simulink library "passive_balancing_plant_lib"  (R2022b)
settings: Solver=VariableStepAuto  StartTime=0.0  StopTime=10.0  RelTol=1e-3
values from neighbouring files (symbols this model uses):
  C1_LUT = 2887.70299486401 4322.85637783158 4303.63777361549 5660.4257619161 10025.6228486411 10795.3803188661 8403.2926645088 10303.8261927401 8639.27645423926 9127.81465902188 33086.4103910671 13371.3754375743 9514.85903729136 34662.1679971819 8026.84086107818 27790.9287411121 14186.8877450726 12734.2960214805 11929.7824894044 12691.2600304428 4549.5148639253 79281.9214895882 7004.71125363224 35331.898561    [passive_balancing_data.sldd]
  Capacity_LUT : value not decoded    [passive_balancing_data.sldd]
  cell_area = 0.1019    [passive_balancing_data.sldd]
  cell_Cp_heat = 964.92    [passive_balancing_data.sldd]
  cell_mass = 0.84    [passive_balancing_data.sldd]
  Em_LUT = 3.48407194875853 3.55418080716149 3.6044040443123 3.64321489304947 3.68502177847119 3.74422605890089 3.82967867350671 3.94315917033962 4.05943812577673 4.19049029477082 3.49373906253632 3.5525957055852 3.61410230902054 3.64896659680084 3.68864192779988 3.74398921633946 3.83940080415011 3.94854312702762 4.06094828281537 4.19030181290971 3.50592874552606 3.55508312112845 3.61515360383738 3.656857038    [passive_balancing_data.sldd]
  h_conv = 5.0    [passive_balancing_data.sldd]
  initial_SOC : value not decoded    [passive_balancing_data.sldd]
  initial_temperature = 293.15    [passive_balancing_data.sldd]
  R0_LUT = 0.0164025520353838 0.0119600956597842 0.0119853068610826 0.0111330643324705 0.011822289585725 0.0116748342939053 0.0112768580015193 0.0118933795996695 0.0120321348242062 0.0124098156482057 0.00991391593917779 0.00875043635238341 0.00832297953681552 0.00872061850253288 0.00795909444960185 0.00856548056926203 0.00843330788647423 0.00850334186162495 0.00846602435735512 0.00846539753229566 0.009331684    [passive_balancing_data.sldd]
  R1_LUT = 0.00470517937000299 0.00290275050725254 0.00173884757466172 0.00166867739185738 0.000922417169458259 0.00120601315196432 0.00134107014418335 0.00102728323615524 0.0010711264474031 0.00109762911159868 0.000293638394729167 0.00090641529499803 0.001265081388855 0.000314621823867429 0.00115254740207724 0.000484496431848577 0.000722662778209487 0.000788593565891369 0.000808964645885711 0.00079463216317    [passive_balancing_data.sldd]
  SOC_LUT : value not decoded    [passive_balancing_data.sldd]
  Temperature_LUT : value not decoded    [passive_balancing_data.sldd]
settings Model: Creator=tshintai  LastModifiedBy=tshintai
settings DebuggingCC: UnconnectedInputMsg=warning  UnconnectedOutputMsg=warning  UnconnectedLineMsg=warning
settings ModelReferenceCC: EnableRefExpFcnMdlSchedulingChecks=on
settings RTWCC: DLArmComputeVersion=19.05

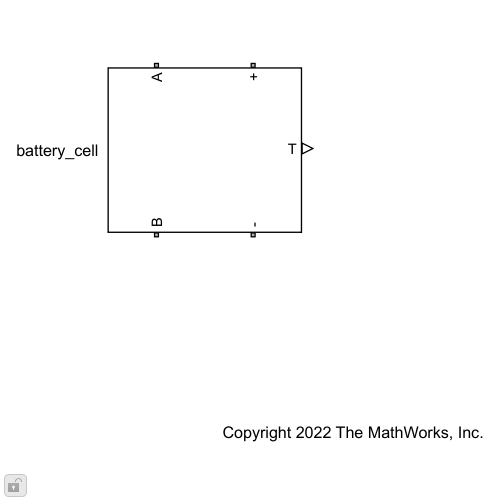
[thumbnail: Simulink's stored preview of the top-level diagram]
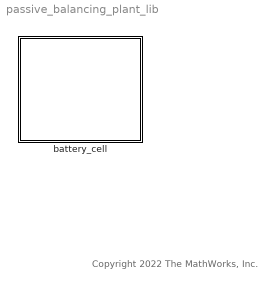
== system passive_balancing_plant_lib ==
  note: Copyright 2022 The MathWorks, Inc.
  battery_cell : Subsystem  mask{SOC_LUT=SOC_LUT, Temperature_LUT=Temperature_LUT, Em_LUT=Em_LUT, R0_LUT=R0_LUT, Capacity_LUT=Capacity_LUT, R1_LUT=R1_LUT, C1_LUT=C1_LUT, cell_mass=cell_mass, cell_Cp_heat=cell_Cp_heat, initial_SOC=initial_SOC, initial_temperature=initial_temperature, cell_area=cell_area, h_conv=h_conv}
      mask prompts: SOC_LUT "SOCのベクトル"; Temperature_LUT "温度のベクトル"; Em_LUT "無負荷電圧"; R0_LUT "端子抵抗R0"; Capacity_LUT "アンペア時評価"; R1_LUT "1番目の分極抵抗R1"; C1_LUT "1 番目のキャパシタンスC1"; cell_mass "セル質量"; cell_Cp_heat "セル熱容量"; initial_SOC "初期SOC"; initial_temperature "初期温度"; cell_area "面積"; h_conv "熱伝達係数"
      settings: PortSchema="{\"entries\":[{\"content\":{\"sides\":[{\"content\":{\"connectorIds\":[]},\"type\":\"ConnectorPlacement.EquallySpacedRectSide\",\"uuid\":\"7476130e-6a6f-4d7d-b81b-0434faf25ed7\"},{\"content\":{\"connectorIds\":[\"RConn1\"],\"side\":\"RIGHT\"},\"type\":\"ConnectorPlacement.EquallySpacedRectSide\",\"uuid\":\"e77f8bc1-535b-4ad6-9f3a-019b907c69f5\"},{\"content\":{\"connectorIds\":[\"LConn1\",\"LConn2\"],\"side\":\"TOP\"},\"type\":\"ConnectorPlacement.EquallySpacedRectSide\",\"uuid\":\"2a79cf03-2226-40db-8021-0cdad01384e5\"},{\"content\":{\"connectorIds\":[\"RConn2\",\"RConn3\"],\"side\":\"BOTTOM\"},\"type\":\"ConnectorPlacement.EquallySpacedRectSide\",\"uuid\":\"ceafb156-d747-4574-a770-c95fd7e4b99a\"}]},\"type\":\"ConnectorPlacement.EquallySpacedConnector\",\"uuid\":\"bdc27146-c1e4-4392-aa17-cfd78a6733fc\"}],\"packageUris\":[\"http://schema.mathworks.com/mf0/Connector/R2020b\"],\"version\":\"1.0\"}"

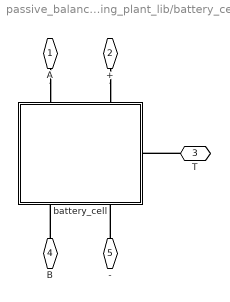
== system passive_balancing_plant_lib/battery_cell ==
  battery_cell : Subsystem  ReferencedSubsystem=Battery_Cell
      settings: PortSchema="{\"entries\":[{\"content\":{\"sides\":[{\"content\":{\"connectorIds\":[]},\"type\":\"ConnectorPlacement.EquallySpacedRectSide\",\"uuid\":\"932f6c20-040f-482d-bb64-d9cf996e59f9\"},{\"content\":{\"connectorIds\":[\"RConn1\"],\"side\":\"RIGHT\"},\"type\":\"ConnectorPlacement.EquallySpacedRectSide\",\"uuid\":\"81221056-e63e-4491-ab4b-dcd69fc99e9b\"},{\"content\":{\"connectorIds\":[\"LConn1\",\"LConn2\"],\"side\":\"TOP\"},\"type\":\"ConnectorPlacement.EquallySpacedRectSide\",\"uuid\":\"66ed0f47-5331-4c25-8328-36f3dabcabb7\"},{\"content\":{\"connectorIds\":[\"RConn2\",\"RConn3\"],\"side\":\"BOTTOM\"},\"type\":\"ConnectorPlacement.EquallySpacedRectSide\",\"uuid\":\"683d1b76-8c4e-4b23-9d0f-34a0c32e2c1c\"}]},\"type\":\"ConnectorPlacement.EquallySpacedConnector\",\"uuid\":\"ee8d2d6f-7fde-4ff7-848c-1d562a4210af\"}],\"packageUris\":[\"http://schema.mathworks.com/mf0/Connector/R2020b\"],\"version\":\"1.0\"}"
  A : PMIOPort  Side=Left
  + : PMIOPort  Port=2  Side=Left
  T : PMIOPort  Port=3  Side=Right
  B : PMIOPort  Port=4  Side=Right
  - : PMIOPort  Port=5  Side=Right
  connections:
  A/RConn1 -- battery_cell/LConn1
  +/RConn1 -- battery_cell/LConn2
  B/RConn1 -- battery_cell/RConn2
  -/RConn1 -- battery_cell/RConn3
  T/RConn1 -- battery_cell/RConn1
